simulink model "feedback_harness"  (R2020b)
settings: Solver=FixedStepDiscrete  StartTime=0.0  StopTime=20  FixedStep=T_sample_control  RelTol=1e-3  EnableMultiTasking=on
settings Model: DataDictionary=pid.sldd  ModifiedByFormat=The MathWorks Inc.  PacingRate=0.010000  Creator=The MathWorks, Inc.  LastModifiedBy=The MathWorks Inc.
settings DataIOCC: LimitDataPoints=on  SaveFormat=Array  SaveOutput=off  SaveTime=off  ReturnWorkspaceOutputs=off
settings OptimizationCC: DefaultParameterBehavior=Inlined  EnhancedBackFolding=on  PassReuseOutputArgsAs=Individual arguments  ExpressionDepthLimit=2147483647  OptimizeBlockOrder=speed  DifferentSizesBufferReuse=on  OptimizationCustomize=off  EfficientTunableParamExpr=on
settings DebuggingCC: UnderspecifiedInitializationDetection=Classic  MergeDetectMultiDrivingBlocksExec=none  SolverPrmCheckMsg=warning  ParameterTunabilityLossMsg=error  FcnCallInpInsideContextMsg=warning  StateNameClashWarn=warning  SFUnexpectedBacktrackingDiag=warning  SFNoUnconditionalDefaultTransitionDiag=warning  SFExecutionAtInitializationDiag=none  ArithmeticOperatorsInVariantConditions=warning
settings HardwareCC: ProdBitPerPointer=32  ProdBitPerSizeT=32  ProdBitPerPtrDiffT=32  ProdLargestAtomicInteger=Long  ProdLargestAtomicFloat=Double  ProdWordSize=32  ProdHWDeviceType=ARM Compatible->ARM Cortex-M
settings ModelReferenceCC: PropagateSignalLabelsOutOfModel=off
settings SFSimCC: SimUseLocalCustomCode=off  MATLABDynamicMemAlloc=off  CustomCodeUndefinedFunction=UseInterfaceOnly
settings RTWCC: Description=Embedded Coder  SystemTargetFile=ert.tlc  TemplateMakefile=ert_default_tmf  GenerateReport=on  RTWUseLocalCustomCode=off  LaunchReport=on
settings CodeAppCC: ForceParamTrailComments=on  IgnoreCustomStorageClasses=off  OperatorAnnotations=on  SimulinkDataObjDesc=on  SFDataObjDesc=on  InsertBlockDesc=on
settings ERTTargetCC: GenerateSampleERTMain=on  CodeInterfacePackaging=Reusable function  InlinedParameterPlacement=NonHierarchical  ERTCustomFileTemplate=example_file_process.tlc  ERTFilePackagingFormat=Compact
settings ConfigComp: CovMetricSettings=dw  CovSaveCumulativeToWorkspaceVar=on  CovSaveSingleToWorkspaceVar=on  CovExternalEMLEnable=off  CovSFcnEnable=off

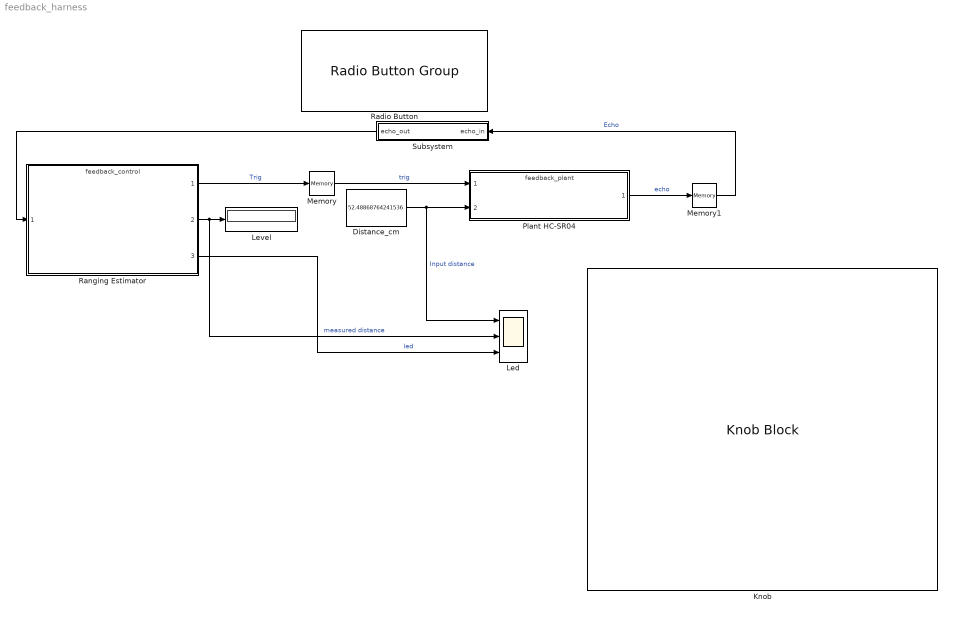
== system feedback_harness ==
  Distance_cm : Constant  Value=52.48868764241536
  Knob : KnobBlock  ScaleMax=410  TickInterval=10
  Led : Scope  NumInputPorts=3
  Level : Display
  Memory : Memory
  Memory1 : Memory
  Plant HC-SR04 : ModelReference  ModelNameDialog=feedback_plant  SimulationMode=Normal  ModelReferenceVersion=10.19
  Radio Button : RadioButtonGroup  SelectedLabel=Sensor Connected  ButtonGroupName=Disconnetion Button
      settings: Values={{'Sensor Disconnected', 'Sensor Connected'}, [0 1]}
  Ranging Estimator : ModelReference  ModelNameDialog=feedback_control  SimulationMode=Normal  ModelReferenceVersion=1.107
  Subsystem : Subsystem
  wires:
  Ranging Estimator/1 -> Memory/1  "Trig"
  Plant HC-SR04/1 -> Memory1/1  "echo"
  Distance_cm/1 -> Led/1, Plant HC-SR04/2  "Input distance"
  Ranging Estimator/3 -> Led/3  "led"
  Memory/1 -> Plant HC-SR04/1  "trig"
  Ranging Estimator/2 -> Led/2, Level/1  "measured distance"
  Memory1/1 -> Subsystem/1(echo_in)  "Echo"
  Subsystem/1(echo_out) -> Ranging Estimator/1

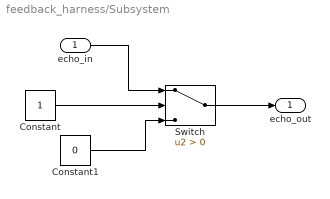
== system feedback_harness/Subsystem ==
  echo_in : Inport  OutDataTypeStr=boolean
  Constant : Constant
  Constant1 : Constant  Value=0  OutDataTypeStr=boolean
  Switch : Switch  Criteria=u2 > Threshold
  echo_out : Outport  OutDataTypeStr=boolean
  wires:
  Constant/1 -> Switch/2
  echo_in/1 -> Switch/1
  Constant1/1 -> Switch/3
  Switch/1 -> echo_out/1
